simulink library "PrachLib"  (R2022a)
settings: Solver=VariableStepAuto  StartTime=0.0  StopTime=10.0  RelTol=1e-3
values from neighbouring files (symbols this model uses):
  ConfigTable = [16 1 9,20,20,20,20,20,20,20,20,20 0 2 6 2 4 ... (first row only)    [ConfigIndexTable.m]
  NTxAnts = 4    [setup_prach_shortFormat.m]    (also in setup_prach_shortFormat_fftShift.m)
undefined symbols (not defined in the file or in its folder): AdvDSPBChannelOutDisplay, AdvDSPBDMemDisplay, display, dpoly, dspba, dspba_ChannelInVis, dspba_ChannelOutVis, dspba_internal_get_channel_ports, evalAionMaskParam, InstanceNumber, latency, PRACH_regs, prach_short, primtype, UseDontCare, value
libraries: DSPBAPrim x280, DSPBAModelBus x7, DSPBAControl x7, $bdroot x3, DspbAdvFftLibrary x1, DSPBAVectorUtil x1
(part 1 of 4)
settings Model: Creator=vmauer  LastModifiedBy=5g
settings SolverCC: AlgebraicLoopSolver=TrustRegion
settings DebuggingCC: UnconnectedInputMsg=warning  UnconnectedOutputMsg=warning  UnconnectedLineMsg=warning  ArithmeticOperatorsInVariantConditions=warning
settings SFSimCC: CustomCodeUndefinedFunction=UseInterfaceOnly

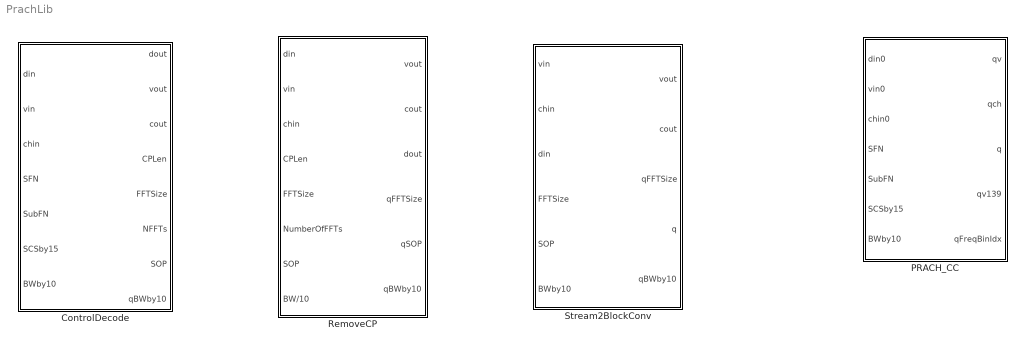
== system PrachLib ==
  ControlDecode : Subsystem  mask{InstanceNumber=InstanceNumber}
      mask prompts: InstanceNumber "CC Index"
  PRACH_CC : Subsystem  mask{InstanceNumber=1}
      mask prompts: InstanceNumber "CC Index"
      mask init:
      | InstanceNumberStr = num2str(InstanceNumber)
      mask Display:
      | color('w');image('dspba_prim.jpg');
      | fprintf('Component\nCarrier\n\n %s\n\nPRACH', int2str(InstanceNumber));
      | port_label('input',1,'din');
      | port_label('input',2,'vin');
      | port_label('input',3,'chin');
      | port_label('input',4,'SFN');
      | port_label('input',5,'SubFN');
      | port_label('input',6,'SCS/15');
      | port_label('input',7,'BW/10');
      | port_label('output',1,'qv');
      | port_label('output',2,'qc');
      | port_label('output',3,'q');
      | port_label('output',4,'qv139');
      | port_label('output',5,'qFFTBinIdx');
  RemoveCP : Subsystem  mask{NAnts=NTxAnts}
      mask prompts: NAnts "Number of Antennas"
  Stream2BlockConv : Subsystem  mask{NAnts=4, NFftMax=prach_short.Nfft}
      mask prompts: NAnts "Number of Antennas"; NFftMax "Maximum FFT size"

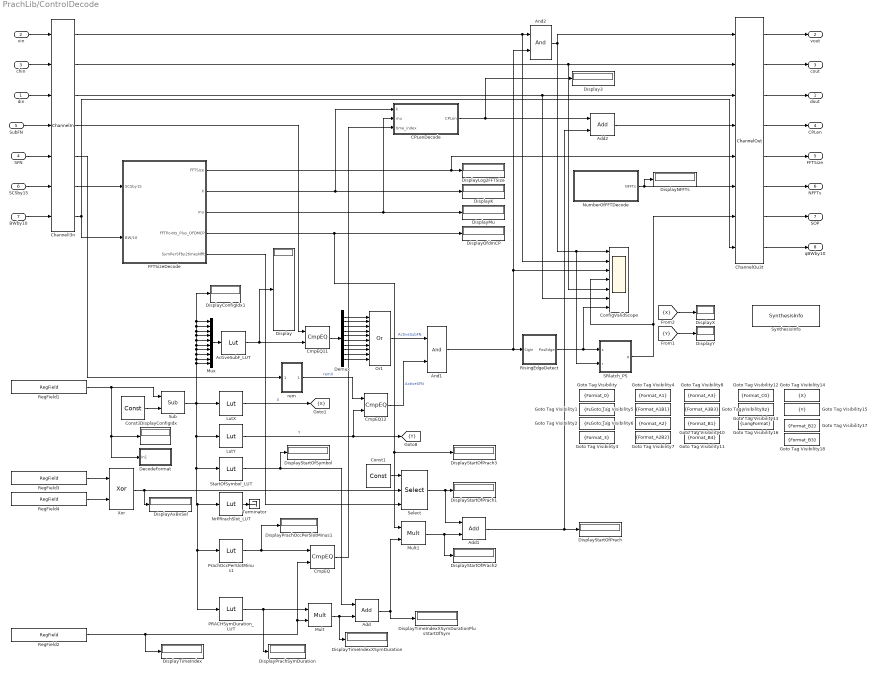
== system PrachLib/ControlDecode ==
  din : Inport
  vin : Inport  Port=2
  chin : Inport  Port=3
  SFN : Inport  Port=4
  SubFN : Inport  Port=5
  SCSby15 : Inport  Port=6
  BWby10 : Inport  Port=7
  ActiveSubF_LUT : DSPBAPrim/Lut  primtype=lut  nInputs=1  nOutputs=1  omode=Inherit via internal rule  otype=sfix(16)  scale=2^-15  rndmethod=Unbiased  factor=1  satmethod=Symmetric  shift_vec=[0 1 2 -1]  value=ConfigTable(:,3:12)  inPortNames=[' '; ' ';]  outPortNames=[' ']  dspbaimage=dspba_prim.svg  text=fprintf('LUT');  style=Optimised  visibilities=8 + 1024  floatPrecision=float32_m23  version=20211007
  Add : DSPBAPrim/Add  primtype=add  nInputs=evalAionMaskParam(gcb,'value',1)  nOutputs=1  omode=Inherit via internal rule with word growth  otype=sfix(16)  scale=2^-15  rndmethod=Unbiased  factor=1  satmethod=Symmetric  shift_vec=[0 1 2 -1]  value=2  inPortNames=[' '; ' ';]  outPortNames=[' ']  dspbaimage=dspba_prim.svg  text=fprintf('+');  style=Optimised  visibilities=1032+2^17+2^18+2^19  genFPC=off  floatRounding=correct  advOptions=[]  version=20211007
  Add1 : DSPBAPrim/Add  primtype=add  nInputs=evalAionMaskParam(gcb,'value',1)  nOutputs=1  omode=Inherit via internal rule with word growth  otype=sfix(16)  scale=2^-15  rndmethod=Unbiased  factor=1  satmethod=Symmetric  shift_vec=[0 1 2 -1]  value=2  inPortNames=[' '; ' ';]  outPortNames=[' ']  dspbaimage=dspba_prim.svg  text=fprintf('+');  style=Optimised  visibilities=1032+2^17+2^18+2^19  genFPC=off  floatRounding=correct  advOptions=[]  version=20211007
  Add2 : DSPBAPrim/Add  primtype=add  nInputs=evalAionMaskParam(gcb,'value',1)  nOutputs=1  omode=Inherit via internal rule with word growth  otype=sfix(16)  scale=2^-15  rndmethod=Unbiased  factor=1  satmethod=Symmetric  shift_vec=[0 1 2 -1]  value=2  inPortNames=[' '; ' ';]  outPortNames=[' ']  dspbaimage=dspba_prim.svg  text=fprintf('+');  style=Optimised  visibilities=1032+2^17+2^18+2^19  genFPC=off  floatRounding=correct  advOptions=[]  version=20211007
  And1 : DSPBAPrim/And  primtype=and  nInputs=2  nOutputs=1  omode=Inherit via internal rule  otype=sfix(16)  scale=2^-15  rndmethod=Unbiased  factor=1  satmethod=Symmetric  shift_vec=[0 1 2 -1]  value=0  inPortNames=[' '; ' '; ' '; ' '; ' '; ' '; ' '; ' '; ' '; ' '; ' '; ' '; ' '; ' '; ' '; ' '; ]  outPortNames=[' ']  dspbaimage=dspba_prim.svg  text=fprintf('&');  style=Optimised  visibilities=8+2  version=20211007
  And2 : DSPBAPrim/And  primtype=and  nInputs=2  nOutputs=1  omode=Inherit via internal rule  otype=sfix(16)  scale=2^-15  rndmethod=Unbiased  factor=1  satmethod=Symmetric  shift_vec=[0 1 2 -1]  value=0  inPortNames=[' '; ' '; ' '; ' '; ' '; ' '; ' '; ' '; ' '; ' '; ' '; ' '; ' '; ' '; ' '; ' '; ]  outPortNames=[' ']  dspbaimage=dspba_prim.svg  text=fprintf('&');  style=Optimised  visibilities=8+2  version=20211007
  CPLenDecode : Subsystem
      mask Display:
      | color('w');
      | image('dspba_prim.jpg');
      | port_label('output',1,'CPLen*nAnt');
      | port_label('input',1,'k');
      | port_label('input',2,'mu');
      | port_label('input',3,'time_index');
  ChannelI3n : DSPBAPrim/ChannelIn  primtype=channelin  nInputs=dspba_internal_get_channel_ports(gcb)  nOutputs=dspba_internal_get_channel_ports(gcb)  omode=Inherit via internal rule  otype=sfix(16)  scale=2^-15  rndmethod=Unbiased  factor=1  satmethod=Symmetric  shift_vec=[0 1 2 -1]  value=5  inPortNames=['v'; 'c'; '0'; '1'; '2'; '3'; '4'; '5'; '6'; '7'; '8'; '9'; 'A'; 'B'; 'D'; 'E'; 'F'; 'G'; 'H'; 'I'; 'J'; 'K'; 'L'; 'M'; 'N'; 'O'; 'P'; 'Q'; 'R'; 'S'; 'T'; 'U'; 'W'; 'X'; 'Y'; 'Z']  outPortNames=['v'; 'c'; '0'; '1'; '2'; '3'; '4'; '5'; '6'; '7'; '8'; '9'; 'A'; 'B'; 'D'; 'E'; 'F'; 'G'; 'H'; 'I'; 'J'; 'K'; 'L'; 'M'; 'N'; 'O'; 'P'; 'Q'; 'R'; 'S'; 'T'; 'U'; 'W'; 'X'; 'Y'; 'Z']  dspbaimage=dspba_prim_channel_tall.svg  text=fprintf('In');  style=Optimised  dataSignals=5  foldingEnabled=off  channels=1  sampleRate=200  packetBeginPresent=off  packetBeginEnabled=off  visibilities=dspba_ChannelInVis(gcb)  latencyCorrection=0  scheduleOrigin=off  version=20211214
  ChannelOu3t : DSPBAPrim/ChannelOut  primtype=channelout  nInputs=dspba_internal_get_channel_ports(gcb)  nOutputs=dspba_internal_get_channel_ports(gcb)  omode=Inherit via internal rule  otype=sfix(16)  scale=2^-15  rndmethod=Unbiased  factor=1  satmethod=Symmetric  shift_vec=[0 1 2 -1]  value=6  inPortNames=['v'; 'c'; '0'; '1'; '2'; '3'; '4'; '5'; '6'; '7'; '8'; '9'; 'A'; 'B'; 'D'; 'E'; 'F'; 'G'; 'H'; 'I'; 'J'; 'K'; 'L'; 'M'; 'N'; 'O'; 'P'; 'Q'; 'R'; 'S'; 'T'; 'U'; 'W'; 'X'; 'Y'; 'Z']  outPortNames=['v'; 'c'; '0'; '1'; '2'; '3'; '4'; '5'; '6'; '7'; '8'; '9'; 'A'; 'B'; 'D'; 'E'; 'F'; 'G'; 'H'; 'I'; 'J'; 'K'; 'L'; 'M'; 'N'; 'O'; 'P'; 'Q'; 'R'; 'S'; 'T'; 'U'; 'W'; 'X'; 'Y'; 'Z']  dspbaimage=dspba_prim_channel_tall.svg  text=fprintf('Out%s', AdvDSPBChannelOutDisplay(latency));  style=Optimised  dataSignals=6  foldingEnabled=off  channels=1  sampleRate=200  packetBeginPresent=off  packetBeginEnabled=off  visibilities=dspba_ChannelOutVis(gcb)  latency=9  latencyCorrection=0  version=20211214
  CmpEQ : DSPBAPrim/CmpEQ  primtype=cmpeq  nInputs=2  nOutputs=1  omode=boolean  otype=sfix(16)  scale=2^-15  rndmethod=Unbiased  factor=1  satmethod=Symmetric  shift_vec=[0 1 2 -1]  value=0  inPortNames=[' '; ' ';]  outPortNames=[' ']  dspbaimage=dspba_prim.svg  text=fprintf('==');  style=Optimised  visibilities=0  advOptions=[]  version=20211007
  CmpEQ11 : DSPBAPrim/CmpEQ  primtype=cmpeq  nInputs=2  nOutputs=1  omode=boolean  otype=sfix(16)  scale=2^-15  rndmethod=Unbiased  factor=1  satmethod=Symmetric  shift_vec=[0 1 2 -1]  value=0  inPortNames=[' '; ' ';]  outPortNames=[' ']  dspbaimage=dspba_prim.svg  text=fprintf('==');  style=Optimised  visibilities=0  advOptions=[]  version=20211007
  CmpEQ12 : DSPBAPrim/CmpEQ  primtype=cmpeq  nInputs=2  nOutputs=1  omode=boolean  otype=sfix(16)  scale=2^-15  rndmethod=Unbiased  factor=1  satmethod=Symmetric  shift_vec=[0 1 2 -1]  value=0  inPortNames=[' '; ' ';]  outPortNames=[' ']  dspbaimage=dspba_prim.svg  text=fprintf('==');  style=Optimised  visibilities=0  advOptions=[]  version=20211007
  ConfigValidScope : Scope  NumInputPorts=7
  Const1 : DSPBAPrim/Const  primtype=const  nInputs=0  nOutputs=1  omode=Inherit via internal rule  otype=sfix(16)  scale=2^-15  rndmethod=Unbiased  factor=1  satmethod=Symmetric  shift_vec=[0 1 2 -1]  value=0  inPortNames=['+'; '+';]  outPortNames=[' ']  dspbaimage=dspba_prim.svg  text=fprintf('%s', num2str(value));  style=Optimised  visibilities=8 + 1024  floatPrecision=float32_m23  warnSaturation=on  version=20211007  SampleTime=inf
  Const3 : DSPBAPrim/Const  primtype=const  nInputs=0  nOutputs=1  omode=Inherit via internal rule  otype=sfix(16)  scale=2^-15  rndmethod=Unbiased  factor=1  satmethod=Symmetric  shift_vec=[0 1 2 -1]  value=67  inPortNames=['+'; '+';]  outPortNames=[' ']  dspbaimage=dspba_prim.svg  text=fprintf('%s', num2str(value));  style=Optimised  visibilities=8 + 1024  floatPrecision=float32_m23  warnSaturation=on  version=20211007  SampleTime=inf
  DecodeFormat : Subsystem
  Demux : Demux  Outputs=10
  Display : Display
  Display3 : Display
  DisplayAxBxSel : Display
  DisplayConfigIdx : Display
  DisplayConfigIdx1 : Display
  DisplayK : Display
  DisplayLog2FFTSize : Display
  DisplayMu : Display
  DisplayNFFTs : Display
  DisplayOfdmCP : Display
  DisplayPrachOccPerSlotMinus1 : Display
  DisplayPrachSymDuration : Display
  DisplayStartOfPrach{,1..3} (4 alike) : Display
  DisplayStartOfSymbol : Display
  DisplayTimeIndex : Display
  DisplayTimeIndexXSymDuration : Display
  DisplayTimeIndexXSymDurationPlusStartOfSym : Display
  DisplayX : Display
  DisplayY : Display
  FFTSizeDecode : Subsystem
      mask Display:
      | color('w');
      | image('dspba_prim.jpg');
      | port_label('output',1,'log2(FFT size)');
      | port_label('output',2,'k');
      | port_label('output',3,'mu');
      | port_label('output',4,'FFTPoints+OFDM_CP');
      | port_label('output',5,'SymPerSF/2*Nfft');
      | port_label('input',1,'SCS/15');
      | port_label('input',2,'BW/10');
  Goto Tag Visibility : GotoTagVisibility  GotoTag=Format_0
  Goto Tag Visibility1 : GotoTagVisibility  GotoTag=Format_1
  Goto Tag Visibility10 : GotoTagVisibility  GotoTag=Format_B1
  Goto Tag Visibility11 : GotoTagVisibility  GotoTag=Format_B4
  Goto Tag Visibility12 : GotoTagVisibility  GotoTag=Format_C0
  Goto Tag Visibility13 : GotoTagVisibility  GotoTag=Format_C2
  Goto Tag Visibility14 : GotoTagVisibility  GotoTag=X
  Goto Tag Visibility15 : GotoTagVisibility  GotoTag=Y
  Goto Tag Visibility16 : GotoTagVisibility  GotoTag=LongFormat
  Goto Tag Visibility17 : GotoTagVisibility  GotoTag=Format_B2
  Goto Tag Visibility18 : GotoTagVisibility  GotoTag=Format_B3
  Goto Tag Visibility2 : GotoTagVisibility  GotoTag=Format_2
  Goto Tag Visibility3 : GotoTagVisibility  GotoTag=Format_3
  Goto Tag Visibility4 : GotoTagVisibility  GotoTag=Format_A1
  Goto Tag Visibility5 : GotoTagVisibility  GotoTag=Format_A1B1
  Goto Tag Visibility6 : GotoTagVisibility  GotoTag=Format_A2
  Goto Tag Visibility7 : GotoTagVisibility  GotoTag=Format_A2B2
  Goto Tag Visibility8 : GotoTagVisibility  GotoTag=Format_A3
  Goto Tag Visibility9 : GotoTagVisibility  GotoTag=Format_A3B3
  LutX : DSPBAPrim/Lut  primtype=lut  nInputs=1  nOutputs=1  omode=Inherit via internal rule  otype=sfix(16)  scale=2^-15  rndmethod=Unbiased  factor=1  satmethod=Symmetric  shift_vec=[0 1 2 -1]  value=ConfigTable(:,1)  inPortNames=[' '; ' ';]  outPortNames=[' ']  dspbaimage=dspba_prim.svg  text=fprintf('LUT');  style=Optimised  visibilities=8 + 1024  floatPrecision=float32_m23  version=20211007
  LutY : DSPBAPrim/Lut  primtype=lut  nInputs=1  nOutputs=1  omode=Inherit via internal rule  otype=sfix(16)  scale=2^-15  rndmethod=Unbiased  factor=1  satmethod=Symmetric  shift_vec=[0 1 2 -1]  value=ConfigTable(:,2)  inPortNames=[' '; ' ';]  outPortNames=[' ']  dspbaimage=dspba_prim.svg  text=fprintf('LUT');  style=Optimised  visibilities=8 + 1024  floatPrecision=float32_m23  version=20211007
  Mult : DSPBAPrim/Mult  primtype=mult  nInputs=2  nOutputs=1  omode=Inherit via internal rule  otype=sfix(16)  scale=2^-15  rndmethod=Unbiased  factor=1  satmethod=Symmetric  shift_vec=[0 1 2 -1]  value=0  inPortNames=[' '; ' ';]  outPortNames=[' ']  dspbaimage=dspba_prim.svg  text=fprintf('X');  style=Optimised  visibilities=8+2^18+2^19  floatPrecision=float32_m23  floatRounding=correct  advOptions=[]  version=20211007
  Mult1 : DSPBAPrim/Mult  primtype=mult  nInputs=2  nOutputs=1  omode=Inherit via internal rule  otype=sfix(16)  scale=2^-15  rndmethod=Unbiased  factor=1  satmethod=Symmetric  shift_vec=[0 1 2 -1]  value=0  inPortNames=[' '; ' ';]  outPortNames=[' ']  dspbaimage=dspba_prim.svg  text=fprintf('X');  style=Optimised  visibilities=8+2^18+2^19  floatPrecision=float32_m23  floatRounding=correct  advOptions=[]  version=20211007
  Mux : Mux  Inputs=10
  NrPRrachSlot_LUT : DSPBAPrim/Lut  primtype=lut  nInputs=1  nOutputs=1  omode=Inherit via internal rule  otype=sfix(16)  scale=2^-15  rndmethod=Unbiased  factor=1  satmethod=Symmetric  shift_vec=[0 1 2 -1]  value=ConfigTable(:,14)  inPortNames=[' '; ' ';]  outPortNames=[' ']  dspbaimage=dspba_prim.svg  text=fprintf('LUT');  style=Optimised  visibilities=8 + 1024  floatPrecision=float32_m23  version=20211007
  NumberOfFFTDecode : Subsystem
      mask Display:
      | color('w');
      | image('dspba_prim.jpg');
      | port_label('output',1,'Number of FFTs');
  Or1 : DSPBAPrim/Or  primtype=or  nInputs=10  nOutputs=1  omode=Inherit via internal rule  otype=sfix(16)  scale=2^-15  rndmethod=Unbiased  factor=1  satmethod=Symmetric  shift_vec=[0 1 2 -1]  value=0  inPortNames=[' '; ' '; ' '; ' '; ' '; ' '; ' '; ' '; ' '; ' '; ' '; ' '; ' '; ' '; ' '; ' '; ]  outPortNames=[' ']  dspbaimage=dspba_prim.svg  text=fprintf('|');  style=Optimised  visibilities=8+2  version=20211007
  PRACHSymDuration_LUT : DSPBAPrim/Lut  primtype=lut  nInputs=1  nOutputs=1  omode=Inherit via internal rule  otype=sfix(16)  scale=2^-15  rndmethod=Unbiased  factor=1  satmethod=Symmetric  shift_vec=[0 1 2 -1]  value=ConfigTable(:,16)  inPortNames=[' '; ' ';]  outPortNames=[' ']  dspbaimage=dspba_prim.svg  text=fprintf('LUT');  style=Optimised  visibilities=8 + 1024  floatPrecision=float32_m23  version=20211007
  PrachOccPerSlotMinus1 : DSPBAPrim/Lut  primtype=lut  nInputs=1  nOutputs=1  omode=Inherit via internal rule  otype=sfix(16)  scale=2^-15  rndmethod=Unbiased  factor=1  satmethod=Symmetric  shift_vec=[0 1 2 -1]  value=ConfigTable(:,15)-1  inPortNames=[' '; ' ';]  outPortNames=[' ']  dspbaimage=dspba_prim.svg  text=fprintf('LUT');  style=Optimised  visibilities=8 + 1024  floatPrecision=float32_m23  version=20211007
  RegField1 : DSPBAModelBus/RegField  reg_name=PRACH_regs(InstanceNumber).PRACH_config_index_addr  reg_rwmode=Read/Write  reg_msb=7  reg_lsb=0  reg_mode=Specify via dialog  reg_type=uint(8)  reg_scale=2^0  reg_init=PRACH_regs(InstanceNumber).PRACH_config_index  reg_desc=PRACH_regs(InstanceNumber).PRACH_config_index_string  reg_modal=off  reg_desc0=0  reg_desc1=0  reg_desc2=0  reg_desc3=0  reg_desc4=0  reg_desc5=0  reg_desc6=0  reg_desc7=0  SampleTime=-1  version=20090407
  RegField2 : DSPBAModelBus/RegField  reg_name=PRACH_regs(InstanceNumber).PRACH_time_index_addr  reg_rwmode=Read/Write  reg_msb=2  reg_lsb=0  reg_mode=Specify via dialog  reg_type=uint(3)  reg_scale=2^0  reg_init=PRACH_regs(InstanceNumber).PRACH_time_index  reg_desc=PRACH_regs(InstanceNumber).PRACH_time_index_string  reg_modal=off  reg_desc0=0  reg_desc1=0  reg_desc2=0  reg_desc3=0  reg_desc4=0  reg_desc5=0  reg_desc6=0  reg_desc7=0  SampleTime=-1  version=20090407
  RegField3 : DSPBAModelBus/RegField  reg_name=PRACH_regs(InstanceNumber).PRACH_NRPRACHSlot_addr  reg_rwmode=Read/Write  reg_msb=0  reg_lsb=0  reg_mode=Specify via dialog  reg_type=uint(1)  reg_scale=2^0  reg_init=PRACH_regs(InstanceNumber).PRACH_NRPRACHSlot  reg_desc=PRACH_regs(InstanceNumber).PRACH_NRPRACHSlot_string  reg_modal=off  reg_desc0=0  reg_desc1=0  reg_desc2=0  reg_desc3=0  reg_desc4=0  reg_desc5=0  reg_desc6=0  reg_desc7=0  SampleTime=-1  version=20090407
  RegField4 : DSPBAModelBus/RegField  reg_name=PRACH_regs(InstanceNumber).PRACH_ActivePRACHSlot_addr  reg_rwmode=Read/Write  reg_msb=0  reg_lsb=0  reg_mode=Specify via dialog  reg_type=uint(1)  reg_scale=2^0  reg_init=PRACH_regs(InstanceNumber).PRACH_ActivePRACHSlot  reg_desc=PRACH_regs(InstanceNumber).PRACH_ActivePRACHSlot_string  reg_modal=off  reg_desc0=0  reg_desc1=0  reg_desc2=0  reg_desc3=0  reg_desc4=0  reg_desc5=0  reg_desc6=0  reg_desc7=0  SampleTime=-1  version=20090407
  RisingEdgeDetect : Subsystem
  SRlatch_PS : Subsystem  AncestorBlock=DSPBAControl/SRlatch_PS  mask(SetResetLatchPrioritySet){}
      mask help: DSP Builder offers two single-cycle latency latch subsystems for common operations for the valid signal, latching with set and reset. The SRlatch block gives priority to the reset input signal; the SRlatch_PS block gives priority to the set input signal. In both blocks, if set and reset inputs are both zero the current output state is maintained.
      mask Help: helpview(dspba.GetHelp('SRlatch_PS'));
      mask Display:
      | color('w');
      | image('dspba_prim_masked.png');
      | fprintf('SRlatch\nPriority\nSet');
      | port_label('input',1,'s');
      | port_label('input',2,'r');
      | port_label('output',1,'q');
  Select : DSPBAPrim/Select  primtype=select  nInputs=str2num(get_param(gcb,'value'))*2+1  nOutputs=1  omode=Inherit via internal rule  otype=sfix(16)  scale=2^-15  rndmethod=Unbiased  factor=1  satmethod=Symmetric  shift_vec=[0 1 2 -1]  value=1  inPortNames=['d'; '0'; 'a'; '1'; 'b'; '2'; 'c'; '3'; 'd'; '4'; 'e'; '5'; 'f'; '6'; 'g'; '7'; 'h'; '8'; 'i'; '9'; 'j']  outPortNames=[' ']  dspbaimage=dspba_prim_tall.svg  text=fprintf('%s', primtype);  style=Optimised  visibilities=8 + 1024  version=20211007
  StartOfSymbol_LUT : DSPBAPrim/Lut  primtype=lut  nInputs=1  nOutputs=1  omode=Inherit via internal rule  otype=sfix(16)  scale=2^-15  rndmethod=Unbiased  factor=1  satmethod=Symmetric  shift_vec=[0 1 2 -1]  value=ConfigTable(:,13)  inPortNames=[' '; ' ';]  outPortNames=[' ']  dspbaimage=dspba_prim.svg  text=fprintf('LUT');  style=Optimised  visibilities=8 + 1024  floatPrecision=float32_m23  version=20211007
  Sub : DSPBAPrim/Sub  primtype=sub  nInputs=2  nOutputs=1  omode=Specify via dialog  otype=uint(8)  scale=1  rndmethod=Unbiased  factor=1  satmethod=Symmetric  shift_vec=[0 1 2 -1]  value=0  inPortNames=['+'; '-';]  outPortNames=[' ']  dspbaimage=dspba_prim.svg  text=fprintf('-');  style=Optimised  visibilities=8+2^17+2^18  floatRounding=correct  advOptions=[]  version=20211007
  SynthesisInfo : DSPBAPrim/SynthesisInfo  primtype=synthinfo  nInputs=0  nOutputs=0  omode=Inherit via internal rule  otype=sfix(16)  scale=2^-15  rndmethod=Truncate  factor=1  satmethod=Symmetric  shift_vec=[0 1 2 -1]  value=99  inPortNames=[' '; ' ';]  outPortNames=[' ']  dspbaimage=dspba_prim_ctrl.jpg  text=fprintf('Style=%s', style);  style=Scheduled  visibilities=2^15+2^17+2^18+2^19  constraintPair=None  constraintRelation=>  constraintLimit=2  modelRefSign=+  modelRef=''  showSchedule=off  simulationMode=Use Global Value  resetMinimization=Conditional - On for ChannelIn/Out only  version=20220106
  Terminator : Terminator
  Xor : DSPBAPrim/Xor  primtype=xor  nInputs=2  nOutputs=1  omode=Inherit via internal rule  otype=sfix(16)  scale=2^-15  rndmethod=Unbiased  factor=1  satmethod=Symmetric  shift_vec=[0 1 2 -1]  value=0  inPortNames=[' '; ' '; ' '; ' '; ' '; ' '; ' '; ' '; ' '; ' '; ' '; ' '; ' '; ' '; ' '; ' '; ]  outPortNames=[' ']  dspbaimage=dspba_prim.svg  text=fprintf('^');  style=Optimised  visibilities=8+2  version=20211007
  rem : Subsystem
  dout : Outport  VectorParamsAs1DForOutWhenUnconnected=off
  vout : Outport  Port=2  VectorParamsAs1DForOutWhenUnconnected=off
  cout : Outport  Port=3  VectorParamsAs1DForOutWhenUnconnected=off
  CPLen : Outport  Port=4  VectorParamsAs1DForOutWhenUnconnected=off
  FFTSize : Outport  Port=5  VectorParamsAs1DForOutWhenUnconnected=off
  NFFTs : Outport  Port=6  VectorParamsAs1DForOutWhenUnconnected=off
  SOP : Outport  Port=7  VectorParamsAs1DForOutWhenUnconnected=off
  qBWby10 : Outport  Port=8  VectorParamsAs1DForOutWhenUnconnected=off
  tag scope: X=scoped, Y=scoped
  wires:
  PrachOccPerSlotMinus1/1 -> DisplayPrachOccPerSlotMinus1/1, CmpEQ/1
  NrPRrachSlot_LUT/1 -> Terminator/1
  CmpEQ/1 -> CPLenDecode/3(time_index)
  SRlatch_PS/1(q) -> ConfigValidScope/4, ChannelOu3t/7
  ChannelOu3t/8 -> qBWby10/1
  Add2/1 -> ChannelOu3t/4
  Add1/1 -> DisplayStartOfPrach/1, Add2/2
  Const1/1 -> Select/1
  Xor/1 -> Select/2, DisplayAxBxSel/1
  Select/1 -> Add1/1, DisplayStartOfPrach1/1
  RegField4/1 -> Xor/2
  RegField3/1 -> Xor/1
  FFTSizeDecode/5(SymPerSFby2timesNfft) -> Select/3
  Mult1/1 -> Add1/2, DisplayStartOfPrach2/1
  Add/1 -> DisplayTimeIndexXSymDurationPlusStartOfSym/1, Mult1/2
  StartOfSymbol_LUT/1 -> Add/1, DisplayStartOfSymbol/1
  Mult/1 -> Add/2, DisplayTimeIndexXSymDuration/1
  PRACHSymDuration_LUT/1 -> Mult/1, DisplayPrachSymDuration/1
  RegField2/1 -> Mult/2, CmpEQ/2, DisplayTimeIndex/1
  FFTSizeDecode/4(FFTPoints_Plus_OFDMCP) -> DisplayOfdmCP/1, DisplayStartOfPrach3/1, Mult1/1
  FFTSizeDecode/1(FFTSize) -> ChannelOu3t/5, DisplayLog2FFTSize/1
  RisingEdgeDetect/1(PosEdge) -> SRlatch_PS/1(s), ConfigValidScope/7
  ChannelOu3t/7 -> SOP/1
  Or1/1 -> And1/1  "ActiveSubFN"
  And1/1 -> ConfigValidScope/3, And2/2, RisingEdgeDetect/1(SigIn)
  ChannelOu3t/6 -> NFFTs/1
  NumberOfFFTDecode/1(NFFTs) -> ChannelOu3t/6, DisplayNFFTs/1
  [Y] -> DisplayY/1
  [X] -> DisplayX/1
  FFTSizeDecode/3(mu) -> DisplayMu/1, CPLenDecode/2(mu)
  FFTSizeDecode/2(k) -> DisplayK/1, CPLenDecode/1(k)
  ChannelI3n/7 -> ChannelOu3t/8, FFTSizeDecode/2(BW/10)
  ChannelI3n/6 -> FFTSizeDecode/1(SCSby15)
  BWby10/1 -> ChannelI3n/7
  SCSby15/1 -> ChannelI3n/6
  ChannelOu3t/5 -> FFTSize/1
  ChannelOu3t/4 -> CPLen/1
  CPLenDecode/1(CPLen) -> Display3/1, Add2/1
  SFN/1 -> ChannelI3n/5
  SubFN/1 -> ChannelI3n/4
  Const3/1 -> Sub/2
  Sub/1 -> Mux/10, Mux/9, Mux/8, Mux/7, Mux/6, Mux/5, Mux/4, Mux/3, Mux/2, Mux/1, DisplayConfigIdx1/1, LutY/1, StartOfSymbol_LUT/1, NrPRrachSlot_LUT/1, PrachOccPerSlotMinus1/1, PRACHSymDuration_LUT/1, LutX/1
  CmpEQ11/1 -> Demux/1
  Demux/10 -> Or1/10
  Demux/9 -> Or1/9
  Demux/8 -> Or1/8
  Demux/7 -> Or1/7
  Demux/6 -> Or1/6
  Demux/5 -> Or1/5
  Demux/4 -> Or1/4
  Demux/3 -> Or1/3
  Demux/2 -> Or1/2
  Demux/1 -> Or1/1
  And2/1 -> ChannelOu3t/1, ConfigValidScope/1, SRlatch_PS/2(r)
  CmpEQ12/1 -> And1/2  "ActiveSFN"
  rem/1(rem) -> CmpEQ12/1  "remX"
  ChannelI3n/5 -> rem/1(SFN)
  RegField1/1 -> Sub/1, DecodeFormat/1(In1), DisplayConfigIdx/1
  ChannelI3n/1 -> And2/1, ConfigValidScope/2
  ChannelOu3t/1 -> vout/1
  ChannelOu3t/2 -> cout/1
  ChannelOu3t/3 -> dout/1
  ChannelI3n/2 -> ConfigValidScope/5, ChannelOu3t/2
  vin/1 -> ChannelI3n/1
  chin/1 -> ChannelI3n/2
  din/1 -> ChannelI3n/3
  ChannelI3n/4 -> CmpEQ11/1
  ChannelI3n/3 -> ChannelOu3t/3, ConfigValidScope/6
  ActiveSubF_LUT/1 -> Display/1, CmpEQ11/2
  Mux/1 -> ActiveSubF_LUT/1
  LutX/1 -> [X]  "X"
  LutY/1 -> CmpEQ12/2, [Y]  "Y"

== system PrachLib/PRACH_CC ==
  din0 : Inport
  vin0 : Inport  Port=2
  chin0 : Inport  Port=3
  SFN : Inport  Port=4
  SubFN : Inport  Port=5
  SCSby15 : Inport  Port=6
  BWby10 : Inport  Port=7
  ControlDecode : $bdroot/ControlDecode  InstanceNumber=InstanceNumber
      link override ChannelI3n: packetBeginEnabled=off  value=5
      link override ChannelOu3t: packetBeginEnabled=off  value=6  latency=0
      link override RegField1: reg_addr=8
      link override RegField2: reg_addr=9
      link override RegField3: reg_addr=10
      link override RegField4: reg_addr=11
  RemoveCP : $bdroot/RemoveCP  NAnts=NTxAnts
  ScaleAndSelect : Subsystem
  Stream2BlockConv : $bdroot/Stream2BlockConv  NAnts=4  NFftMax=prach_short.Nfft
  VFFT : Subsystem  AncestorBlock=DspbAdvFftLibrary/Common/VFFT  Opaque=on  mask{IFFT=false, subchannels=1, br_in=true, maxSize=log2(prach_short.Nfft), minSize=9, in_type=prach_short.InputType, type_strings=prach_short.type_strings, faithful=false}
      mask prompts: subchannels "Number of interleaved subchannels (must be a power of 2)"; br_in "Bit-reversed input"; maxSize "maxSize, where the (I)FFT has at most 2^maxSize points"; minSize "minSize, where the (I)FFT has at least 2^minSize points"; in_type "Input type"; type_strings "Twiddle/pruning specification"; faithful "Use faithful rounding"
      mask init:
      | block = gcb;
      | 
      | % Check that we have a legal number of subchannels
      | subchannelbits = ceil(log2(subchannels));
      | if not(subchannels == 2^subchannelbits)
      |     error('%s: subchannels count %d is not a power of 2', block, subchannels);
      | end
      | 
      | if IFFT
      |     FFTstring = 'IFFT';
      | else
      |     FFTstring = 'FFT';
      | end
      | 
      | if br_in
      |     directionString = 'BR->NAT';
      | else
      |     directionString = 'NAT->BR';
      | end
      | 
      | if 1 < subchannels
      |     subchannelString = sprintf('%d subchannels',subchannels);
      | else
      |     subchannelString = '';
      | end
      mask Help: helpview(dspba.GetHelp('fft'));
      mask Display:
      | color('w');
      | image('dspba_fft.jpg');
      | port_label('input',1,'v');
      | port_label('input',2,'c');
      | port_label('input',3,'size');
      | port_label('input',4,'d');
      | port_label('input',5,'BW/10');
      | port_label('output',1,'qv');
      | port_label('output',2,'qc');
      | port_label('output',3,'qsize');
      | port_label('output',4,'q');
      | port_label('output',5,'qBW/10');
      | text(0.30,0.65,sprintf('V%s Core',FFTstring));
      | text(0.35,0.55,sprintf('2^{%d} to 2^{%d}',minSize,maxSize),'texmode','on');
      | text(0.30,0.45,directionString);
      | text(0.20,0.30,subchannelString);
  qv : Outport
  qch : Outport  Port=2
  q : Outport  Port=3
  qv139 : Outport  Port=4
  qFreqBinIdx : Outport  Port=5
  wires:
  SFN/1 -> ControlDecode/4
  din0/1 -> ControlDecode/1
  SubFN/1 -> ControlDecode/5
  chin0/1 -> ControlDecode/3
  vin0/1 -> ControlDecode/2
  BWby10/1 -> ControlDecode/7
  SCSby15/1 -> ControlDecode/6
  RemoveCP/2 -> Stream2BlockConv/2
  RemoveCP/1 -> Stream2BlockConv/1
  RemoveCP/3 -> Stream2BlockConv/3
  RemoveCP/4 -> Stream2BlockConv/4
  RemoveCP/5 -> Stream2BlockConv/5
  VFFT/1(qv) -> ScaleAndSelect/1(vin)
  VFFT/2(qc) -> ScaleAndSelect/2(chin)
  VFFT/3(qsize) -> ScaleAndSelect/3(FFTSize)
  VFFT/4(q) -> ScaleAndSelect/4(d)
  ScaleAndSelect/1(qv) -> qv/1
  ScaleAndSelect/2(qch) -> qch/1
  ScaleAndSelect/3(q) -> q/1
  ScaleAndSelect/4(qv139) -> qv139/1
  ScaleAndSelect/5(FreqBinIdx) -> qFreqBinIdx/1
  RemoveCP/6 -> Stream2BlockConv/6
  Stream2BlockConv/5 -> VFFT/5(BWby10)
  VFFT/5(qBWby10) -> ScaleAndSelect/5(BWby10)
  Stream2BlockConv/1 -> VFFT/1(v)
  Stream2BlockConv/2 -> VFFT/2(c)
  Stream2BlockConv/3 -> VFFT/3(size)
  Stream2BlockConv/4 -> VFFT/4(d)
  ControlDecode/1 -> RemoveCP/1
  ControlDecode/2 -> RemoveCP/2
  ControlDecode/3 -> RemoveCP/3
  ControlDecode/4 -> RemoveCP/4
  ControlDecode/5 -> RemoveCP/5
  ControlDecode/6 -> RemoveCP/6
  ControlDecode/7 -> RemoveCP/7
  ControlDecode/8 -> RemoveCP/8

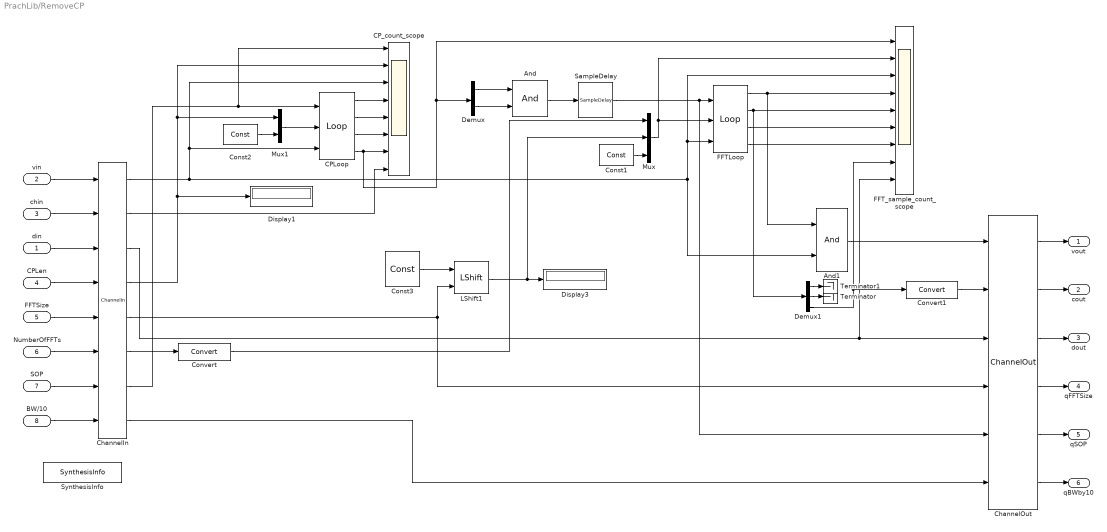
== system PrachLib/RemoveCP ==
  din : Inport
  vin : Inport  Port=2
  chin : Inport  Port=3
  CPLen : Inport  Port=4
  FFTSize : Inport  Port=5
  NumberOfFFTs : Inport  Port=6
  SOP : Inport  Port=7
  BW/10 : Inport  Port=8
  And : DSPBAPrim/And  primtype=and  nInputs=2  nOutputs=1  omode=Inherit via internal rule  otype=sfix(16)  scale=2^-15  rndmethod=Unbiased  factor=1  satmethod=Symmetric  shift_vec=[0 1 2 -1]  value=0  inPortNames=[' '; ' '; ' '; ' '; ' '; ' '; ' '; ' '; ' '; ' '; ' '; ' '; ' '; ' '; ' '; ' '; ]  outPortNames=[' ']  dspbaimage=dspba_prim.svg  text=fprintf('&');  style=Optimised  visibilities=8+2  version=20211007
  And1 : DSPBAPrim/And  primtype=and  nInputs=2  nOutputs=1  omode=Inherit via internal rule  otype=sfix(16)  scale=2^-15  rndmethod=Unbiased  factor=1  satmethod=Symmetric  shift_vec=[0 1 2 -1]  value=0  inPortNames=[' '; ' '; ' '; ' '; ' '; ' '; ' '; ' '; ' '; ' '; ' '; ' '; ' '; ' '; ' '; ' '; ]  outPortNames=[' ']  dspbaimage=dspba_prim.svg  text=fprintf('&');  style=Optimised  visibilities=8+2  version=20211007
  CPLoop : DSPBAPrim/Loop  primtype=loop  nInputs=3  nOutputs=4  omode=Inherit via internal rule  otype=sfix(16)  scale=2^-15  rndmethod=Unbiased  factor=1  satmethod=Symmetric  shift_vec=[0 1 2 -1]  value=[zeros(16, 1)]  inPortNames=['g'; 'c'; 'e']  outPortNames=['v'; 'q'; 'f'; 'l']  dspbaimage=dspba_prim_tall.svg  text=fprintf('loop');  style=Optimised  visibilities=0  version=20211007
  CP_count_scope : Scope  NumInputPorts=8
  ChannelIn : DSPBAPrim/ChannelIn  primtype=channelin  nInputs=dspba_internal_get_channel_ports(gcb)  nOutputs=dspba_internal_get_channel_ports(gcb)  omode=Inherit via internal rule  otype=sfix(16)  scale=2^-15  rndmethod=Unbiased  factor=1  satmethod=Symmetric  shift_vec=[0 1 2 -1]  value=6  inPortNames=['v'; 'c'; '0'; '1'; '2'; '3'; '4'; '5'; '6'; '7'; '8'; '9'; 'A'; 'B'; 'D'; 'E'; 'F'; 'G'; 'H'; 'I'; 'J'; 'K'; 'L'; 'M'; 'N'; 'O'; 'P'; 'Q'; 'R'; 'S'; 'T'; 'U'; 'W'; 'X'; 'Y'; 'Z']  outPortNames=['v'; 'c'; '0'; '1'; '2'; '3'; '4'; '5'; '6'; '7'; '8'; '9'; 'A'; 'B'; 'D'; 'E'; 'F'; 'G'; 'H'; 'I'; 'J'; 'K'; 'L'; 'M'; 'N'; 'O'; 'P'; 'Q'; 'R'; 'S'; 'T'; 'U'; 'W'; 'X'; 'Y'; 'Z']  dspbaimage=dspba_prim_channel_tall.svg  text=fprintf('In');  style=Optimised  dataSignals=6  foldingEnabled=off  channels=1  sampleRate=200  packetBeginPresent=off  packetBeginEnabled=off  visibilities=dspba_ChannelInVis(gcb)  latencyCorrection=0  scheduleOrigin=off  version=20211214
  ChannelOut : DSPBAPrim/ChannelOut  primtype=channelout  nInputs=dspba_internal_get_channel_ports(gcb)  nOutputs=dspba_internal_get_channel_ports(gcb)  omode=Inherit via internal rule  otype=sfix(16)  scale=2^-15  rndmethod=Unbiased  factor=1  satmethod=Symmetric  shift_vec=[0 1 2 -1]  value=4  inPortNames=['v'; 'c'; '0'; '1'; '2'; '3'; '4'; '5'; '6'; '7'; '8'; '9'; 'A'; 'B'; 'D'; 'E'; 'F'; 'G'; 'H'; 'I'; 'J'; 'K'; 'L'; 'M'; 'N'; 'O'; 'P'; 'Q'; 'R'; 'S'; 'T'; 'U'; 'W'; 'X'; 'Y'; 'Z']  outPortNames=['v'; 'c'; '0'; '1'; '2'; '3'; '4'; '5'; '6'; '7'; '8'; '9'; 'A'; 'B'; 'D'; 'E'; 'F'; 'G'; 'H'; 'I'; 'J'; 'K'; 'L'; 'M'; 'N'; 'O'; 'P'; 'Q'; 'R'; 'S'; 'T'; 'U'; 'W'; 'X'; 'Y'; 'Z']  dspbaimage=dspba_prim_channel_tall.svg  text=fprintf('Out%s', AdvDSPBChannelOutDisplay(latency));  style=Optimised  dataSignals=4  foldingEnabled=off  channels=1  sampleRate=200  packetBeginPresent=off  packetBeginEnabled=off  visibilities=dspba_ChannelOutVis(gcb)  latency=0  latencyCorrection=0  version=20211214
  Const1 : DSPBAPrim/Const  primtype=const  nInputs=0  nOutputs=1  omode=Inherit via back propagation  otype=sfix(16)  scale=2^-15  rndmethod=Unbiased  factor=1  satmethod=Symmetric  shift_vec=[0 1 2 -1]  value=NAnts  inPortNames=['+'; '+';]  outPortNames=[' ']  dspbaimage=dspba_prim.svg  text=fprintf('%s', num2str(value));  style=Optimised  visibilities=8 + 1024  floatPrecision=float32_m23  warnSaturation=on  version=20211007  SampleTime=inf
  Const2 : DSPBAPrim/Const  primtype=const  nInputs=0  nOutputs=1  omode=Inherit via back propagation  otype=sfix(16)  scale=2^-15  rndmethod=Unbiased  factor=1  satmethod=Symmetric  shift_vec=[0 1 2 -1]  value=NAnts  inPortNames=['+'; '+';]  outPortNames=[' ']  dspbaimage=dspba_prim.svg  text=fprintf('%s', num2str(value));  style=Optimised  visibilities=8 + 1024  floatPrecision=float32_m23  warnSaturation=on  version=20211007  SampleTime=inf
  Const3 : DSPBAPrim/Const  primtype=const  nInputs=0  nOutputs=1  omode=Inherit via internal rule  otype=sfix(16)  scale=2^-15  rndmethod=Unbiased  factor=1  satmethod=Symmetric  shift_vec=[0 1 2 -1]  value=1  inPortNames=['+'; '+';]  outPortNames=[' ']  dspbaimage=dspba_prim.svg  text=fprintf('%s', num2str(value));  style=Optimised  visibilities=8 + 1024  floatPrecision=float32_m23  warnSaturation=on  version=20211007  SampleTime=inf
  Convert : DSPBAPrim/Convert  primtype=convert  nInputs=1  nOutputs=1  omode=Inherit via back propagation  otype=sfix(16)  scale=2^-15  rndmethod=Truncate  factor=1  satmethod=None  shift_vec=[0 1 2 -1]  value=round([0:255]/17)  inPortNames=[' '; ' ';]  outPortNames=[' '; 'c']  dspbaimage=dspba_prim_wide.svg  text=fprintf('convert');  style=Optimised  visibilities=8+64+256+2^17  clipdetect=off  floatPrecision=float32_m23  advOptions=[]  version=20211007
  Convert1 : DSPBAPrim/Convert  primtype=convert  nInputs=1  nOutputs=1  omode=Specify via dialog  otype=ufix(8)  scale=1  rndmethod=Truncate  factor=1  satmethod=None  shift_vec=[0 1 2 -1]  value=round([0:255]/17)  inPortNames=[' '; ' ';]  outPortNames=[' '; 'c']  dspbaimage=dspba_prim_wide.svg  text=fprintf('convert');  style=Optimised  visibilities=8+64+256+2^17  clipdetect=off  floatPrecision=float32_m23  advOptions=[]  version=20211007
  Demux : Demux  Outputs=2
  Demux1 : Demux  Outputs=3
  Display1 : Display
  Display3 : Display
  FFTLoop : DSPBAPrim/Loop  primtype=loop  nInputs=3  nOutputs=4  omode=Inherit via internal rule  otype=sfix(16)  scale=2^-15  rndmethod=Unbiased  factor=1  satmethod=Symmetric  shift_vec=[0 1 2 -1]  value=[zeros(16, 1)]  inPortNames=['g'; 'c'; 'e']  outPortNames=['v'; 'q'; 'f'; 'l']  dspbaimage=dspba_prim_tall.svg  text=fprintf('loop');  style=Optimised  visibilities=0  version=20211007
  FFT_sample_count_scope : Scope  NumInputPorts=9
  LShift1 : DSPBAPrim/LShift  primtype=lshift  nInputs=2  nOutputs=1  omode=Specify via dialog  otype=ufix(log2(prach_short.Nfft)+1)  scale=1  rndmethod=Unbiased  factor=1  satmethod=Symmetric  shift_vec=[0 1 2 -1]  value=0  inPortNames=['a'; 'b';]  outPortNames=[' ']  dspbaimage=dspba_prim.svg  text=fprintf('a << b');  style=Optimised  visibilities=8  version=20211007
  Mux : Mux  Inputs=3
  Mux1 : Mux  Inputs=2
  SampleDelay : DSPBAPrim/SampleDelay  primtype=sampdelay  nInputs=1  nOutputs=1  omode=Inherit via internal rule  otype=sfix(16)  scale=2^-15  rndmethod=Unbiased  factor=1  satmethod=Symmetric  shift_vec=[0 1 2 -1]  floatPrecision=float32_m23  value=1  inPortNames=[' '; ' ';]  outPortNames=[' ']  dspbaimage=dspba_prim.svg  text=dpoly(1, eye(1,value+1), 'z')  style=Optimised  visibilities=8 + 1024 + 2^17 + 2^18  flexible=off  slackgroup=0  augmented=0  version=20211007  advOptions=[]
  SynthesisInfo : DSPBAPrim/SynthesisInfo  primtype=synthinfo  nInputs=0  nOutputs=0  omode=Inherit via internal rule  otype=sfix(16)  scale=2^-15  rndmethod=Truncate  factor=1  satmethod=Symmetric  shift_vec=[0 1 2 -1]  value=99  inPortNames=[' '; ' ';]  outPortNames=[' ']  dspbaimage=dspba_prim_ctrl.jpg  text=fprintf('Style=%s', style);  style=Scheduled  visibilities=32768  constraintPair=None  constraintRelation=>  constraintLimit=6  modelRefSign=+  modelRef=''  showSchedule=off  simulationMode=Use Global Value  resetMinimization=Conditional - On for ChannelIn/Out only  version=20220106
  Terminator : Terminator
  Terminator1 : Terminator
  vout : Outport  VectorParamsAs1DForOutWhenUnconnected=off
  cout : Outport  Port=2  VectorParamsAs1DForOutWhenUnconnected=off
  dout : Outport  Port=3  VectorParamsAs1DForOutWhenUnconnected=off
  qFFTSize : Outport  Port=4  VectorParamsAs1DForOutWhenUnconnected=off
  qSOP : Outport  Port=5  VectorParamsAs1DForOutWhenUnconnected=off
  qBWby10 : Outport  Port=6  VectorParamsAs1DForOutWhenUnconnected=off
  wires:
  ChannelIn/3 -> FFT_sample_count_scope/9, ChannelOut/3
  Convert1/1 -> ChannelOut/2
  Demux1/2 -> Terminator/1
  Demux1/1 -> Terminator1/1
  Demux1/3 -> FFT_sample_count_scope/8, Convert1/1
  SampleDelay/1 -> FFTLoop/1, ChannelOut/5
  ChannelIn/8 -> ChannelOut/6
  ChannelOut/6 -> qBWby10/1
  BW/10/1 -> ChannelIn/8
  ChannelOut/4 -> qFFTSize/1
  ChannelOut/5 -> qSOP/1
  Demux/1 -> And/1
  Demux/2 -> And/2
  And/1 -> SampleDelay/1
  Const2/1 -> Mux1/2
  Mux1/1 -> CPLoop/2
  Const1/1 -> Mux/3
  Convert/1 -> Mux/1
  LShift1/1 -> Display3/1, Mux/2
  Const3/1 -> LShift1/1
  CPLoop/3 -> CP_count_scope/6
  CPLoop/2 -> CP_count_scope/5
  CPLoop/1 -> CP_count_scope/4
  FFTLoop/4 -> FFT_sample_count_scope/7
  FFTLoop/3 -> FFT_sample_count_scope/6
  FFTLoop/2 -> FFT_sample_count_scope/5, Demux1/1
  CPLoop/4 -> FFT_sample_count_scope/1, Demux/1, CP_count_scope/7
  Mux/1 -> FFTLoop/2, FFT_sample_count_scope/2
  FFTLoop/1 -> FFT_sample_count_scope/4, And1/1
  SOP/1 -> ChannelIn/7
  ChannelIn/7 -> CPLoop/1, CP_count_scope/1
  ChannelIn/4 -> Display1/1, Mux1/1, CP_count_scope/2
  ChannelIn/6 -> Convert/1
  vin/1 -> ChannelIn/1
  din/1 -> ChannelIn/3
  chin/1 -> ChannelIn/2
  NumberOfFFTs/1 -> ChannelIn/6
  ChannelIn/5 -> ChannelOut/4, LShift1/2
  FFTSize/1 -> ChannelIn/5
  CPLen/1 -> ChannelIn/4
  And1/1 -> ChannelOut/1
  ChannelIn/2 -> CP_count_scope/8
  ChannelOut/1 -> vout/1
  ChannelOut/2 -> cout/1
  ChannelOut/3 -> dout/1
  ChannelIn/1 -> And1/2, FFTLoop/3, FFT_sample_count_scope/3, CP_count_scope/3, CPLoop/3

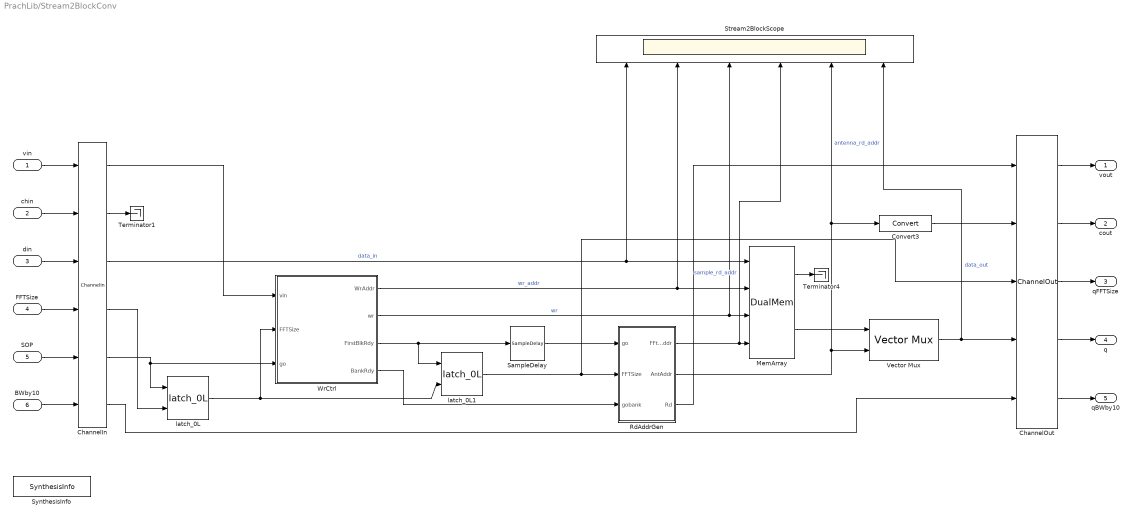
== system PrachLib/Stream2BlockConv ==
  vin : Inport
  chin : Inport  Port=2
  din : Inport  Port=3
  FFTSize : Inport  Port=4
  SOP : Inport  Port=5
  BWby10 : Inport  Port=6
  ChannelIn : DSPBAPrim/ChannelIn  primtype=channelin  nInputs=dspba_internal_get_channel_ports(gcb)  nOutputs=dspba_internal_get_channel_ports(gcb)  omode=Inherit via internal rule  otype=sfix(16)  scale=2^-15  rndmethod=Unbiased  factor=1  satmethod=Symmetric  shift_vec=[0 1 2 -1]  value=4  inPortNames=['v'; 'c'; '0'; '1'; '2'; '3'; '4'; '5'; '6'; '7'; '8'; '9'; 'A'; 'B'; 'D'; 'E'; 'F'; 'G'; 'H'; 'I'; 'J'; 'K'; 'L'; 'M'; 'N'; 'O'; 'P'; 'Q'; 'R'; 'S'; 'T'; 'U'; 'W'; 'X'; 'Y'; 'Z']  outPortNames=['v'; 'c'; '0'; '1'; '2'; '3'; '4'; '5'; '6'; '7'; '8'; '9'; 'A'; 'B'; 'D'; 'E'; 'F'; 'G'; 'H'; 'I'; 'J'; 'K'; 'L'; 'M'; 'N'; 'O'; 'P'; 'Q'; 'R'; 'S'; 'T'; 'U'; 'W'; 'X'; 'Y'; 'Z']  dspbaimage=dspba_prim_channel_tall.svg  text=fprintf('In');  style=Optimised  dataSignals=4  foldingEnabled=off  channels=1  sampleRate=200  packetBeginPresent=off  packetBeginEnabled=off  visibilities=dspba_ChannelInVis(gcb)  latencyCorrection=0  scheduleOrigin=off  version=20211214
  ChannelOut : DSPBAPrim/ChannelOut  primtype=channelout  nInputs=dspba_internal_get_channel_ports(gcb)  nOutputs=dspba_internal_get_channel_ports(gcb)  omode=Inherit via internal rule  otype=sfix(16)  scale=2^-15  rndmethod=Unbiased  factor=1  satmethod=Symmetric  shift_vec=[0 1 2 -1]  value=3  inPortNames=['v'; 'c'; '0'; '1'; '2'; '3'; '4'; '5'; '6'; '7'; '8'; '9'; 'A'; 'B'; 'D'; 'E'; 'F'; 'G'; 'H'; 'I'; 'J'; 'K'; 'L'; 'M'; 'N'; 'O'; 'P'; 'Q'; 'R'; 'S'; 'T'; 'U'; 'W'; 'X'; 'Y'; 'Z']  outPortNames=['v'; 'c'; '0'; '1'; '2'; '3'; '4'; '5'; '6'; '7'; '8'; '9'; 'A'; 'B'; 'D'; 'E'; 'F'; 'G'; 'H'; 'I'; 'J'; 'K'; 'L'; 'M'; 'N'; 'O'; 'P'; 'Q'; 'R'; 'S'; 'T'; 'U'; 'W'; 'X'; 'Y'; 'Z']  dspbaimage=dspba_prim_channel_tall.svg  text=fprintf('Out%s', AdvDSPBChannelOutDisplay(latency));  style=Optimised  dataSignals=3  foldingEnabled=off  channels=1  sampleRate=200  packetBeginPresent=off  packetBeginEnabled=off  visibilities=dspba_ChannelOutVis(gcb)  latency=0  latencyCorrection=0  version=20211214
  Convert3 : DSPBAPrim/Convert  primtype=convert  nInputs=1  nOutputs=1  omode=Specify via dialog  otype=uint(8)  scale=1  rndmethod=Truncate  factor=1  satmethod=None  shift_vec=[0 1 2 -1]  value=round([0:255]/17)  inPortNames=[' '; ' ';]  outPortNames=[' '; 'c']  dspbaimage=dspba_prim_wide.svg  text=fprintf('convert');  style=Optimised  visibilities=8+64+256+2^17  clipdetect=off  floatPrecision=float32_m23  advOptions=[]  version=20211007
  MemArray : DSPBAPrim/DualMem  primtype=dualmem  nInputs=4  nOutputs=2  omode=Inherit via internal rule  otype=sfix(16)  scale=2^-15  rndmethod=Unbiased  factor=1  satmethod=Symmetric  shift_vec=[0 1 2 -1]  value=[zeros(NFftMax*2, NAnts)]  inPortNames=['d1'; 'a1'; 'w1'; 'a2']  outPortNames=['q1'; 'q2']  dspbaimage=dspba_prim_tall.svg  text=fprintf('dmem%s',AdvDSPBDMemDisplay(UseDontCare));  style=Optimised  visibilities=8 + 1024 + 2^17 + 2^18  UseDontCare=on  TwinWritePorts=off  init=on  ProvideReadAccess=off  version=20211007
  RdAddrGen : Subsystem  mask{NAnts=NAnts, NFftMax=NFftMax}
      mask prompts: NAnts "Number of Antennas"; NFftMax "Maximum FFT size"
  SampleDelay : DSPBAPrim/SampleDelay  primtype=sampdelay  nInputs=1  nOutputs=1  omode=Inherit via internal rule  otype=sfix(16)  scale=2^-15  rndmethod=Unbiased  factor=1  satmethod=Symmetric  shift_vec=[0 1 2 -1]  floatPrecision=float32_m23  value=1  inPortNames=[' '; ' ';]  outPortNames=[' ']  dspbaimage=dspba_prim.svg  text=dpoly(1, eye(1,value+1), 'z')  style=Optimised  visibilities=8 + 1024 + 2^17 + 2^18  flexible=off  slackgroup=0  augmented=0  version=20211007  advOptions=[]
  Stream2BlockScope : Scope  NumInputPorts=6
  SynthesisInfo : DSPBAPrim/SynthesisInfo  primtype=synthinfo  nInputs=0  nOutputs=0  omode=Inherit via internal rule  otype=sfix(16)  scale=2^-15  rndmethod=Truncate  factor=1  satmethod=Symmetric  shift_vec=[0 1 2 -1]  value=99  inPortNames=[' '; ' ';]  outPortNames=[' ']  dspbaimage=dspba_prim_ctrl.jpg  text=fprintf('Style=%s', style);  style=Scheduled  visibilities=32768  constraintPair=None  constraintRelation=>  constraintLimit=6  modelRefSign=+  modelRef=''  showSchedule=off  simulationMode=Use Global Value  resetMinimization=Conditional - On for ChannelIn/Out only  version=20220106
  Terminator1 : Terminator
  Terminator4 : Terminator
  Vector Mux : DSPBAVectorUtil/Vector Mux  vecWidth=NAnts
  WrCtrl : Subsystem  mask{NAnts=NAnts, NFftMax=NFftMax}
      mask prompts: NAnts "Number of Antennas"; NFftMax "Maximum FFT size"
  latch_0L : DSPBAControl/latch_0L
  latch_0L1 : DSPBAControl/latch_0L
  vout : Outport  VectorParamsAs1DForOutWhenUnconnected=off
  cout : Outport  Port=2  VectorParamsAs1DForOutWhenUnconnected=off
  qFFTSize : Outport  Port=3  VectorParamsAs1DForOutWhenUnconnected=off
  q : Outport  Port=4  VectorParamsAs1DForOutWhenUnconnected=off
  qBWby10 : Outport  Port=5  VectorParamsAs1DForOutWhenUnconnected=off
  wires:
  WrCtrl/4(BankRdy) -> RdAddrGen/3(gobank)
  SampleDelay/1 -> RdAddrGen/1(go)
  ChannelIn/6 -> ChannelOut/5
  ChannelOut/5 -> qBWby10/1
  BWby10/1 -> ChannelIn/6
  ChannelOut/4 -> q/1
  ChannelOut/3 -> qFFTSize/1
  ChannelIn/5 -> latch_0L/1, WrCtrl/3(go)
  ChannelIn/4 -> latch_0L/2
  SOP/1 -> ChannelIn/5
  FFTSize/1 -> ChannelIn/4
  ChannelIn/2 -> Terminator1/1
  RdAddrGen/3(Rd) -> ChannelOut/1
  WrCtrl/3(FirstBlkRdy) -> SampleDelay/1, latch_0L1/1
  WrCtrl/2(wr) -> Stream2BlockScope/3, MemArray/3  "wr"
  WrCtrl/1(WrAddr) -> Stream2BlockScope/2, MemArray/2  "wr_addr"
  Convert3/1 -> ChannelOut/2
  RdAddrGen/1(FFtPntAddr) -> Stream2BlockScope/4, MemArray/4  "sample_rd_addr"
  latch_0L1/1 -> RdAddrGen/2(FFTSize), ChannelOut/3
  latch_0L/1 -> latch_0L1/2, WrCtrl/2(FFTSize)
  MemArray/1 -> Terminator4/1
  Vector Mux/1 -> Stream2BlockScope/6, ChannelOut/4  "data_out"
  MemArray/2 -> Vector Mux/1
  ChannelIn/3 -> Stream2BlockScope/1, MemArray/1  "data_in"
  RdAddrGen/2(AntAddr) -> Stream2BlockScope/5, Convert3/1, Vector Mux/2  "antenna_rd_addr"
  ChannelIn/1 -> WrCtrl/1(vin)
  din/1 -> ChannelIn/3
  chin/1 -> ChannelIn/2
  vin/1 -> ChannelIn/1
  ChannelOut/2 -> cout/1
  ChannelOut/1 -> vout/1
